simulink model "TorqueControl"  (R2022a)
settings: Solver=FixedStepAuto  StartTime=0.0  StopTime=inf  FixedStep=.001  RelTol=1e-3  EnableMultiTasking=on
undefined symbols (not defined in the file): DiscIntNeverNeededParam
libraries: simulink x7, slrealtimeutilitieslib x3, slrealtimeseriallib x2, slrealtimeloglib x2, eeGeneralControl x1
settings Model: sg_rtwmakecfg_data=_sg_IO75X_v1_2_0__sg_netxLib_MSVC140_  SimulationMode=external  ExtModeEnableFloating=off  Creator=a.beck  LastModifiedBy=Jason
settings SolverCC: ConcurrentTasks=on  AlgebraicLoopSolver=TrustRegion  PositivePriorityOrder=on  AutoInsertRateTranBlk=on  InsertRTBMode=Never (minimum delay)
settings DataIOCC: LimitDataPoints=on  SaveFormat=StructureWithTime  ReturnWorkspaceOutputs=off
settings OptimizationCC: BlockReduction=off  BooleanDataType=off  OptimizeBlockIOStorage=off  BufferReuse=off  GlobalBufferReuse=off  ExpressionFolding=off  LocalBlockOutputs=off  OptimizeDataStoreBuffers=off  BusAssignmentInplaceUpdate=off
settings DebuggingCC: SaveWithParameterizedLinksMsg=none  UnderspecifiedInitializationDetection=Classic  MergeDetectMultiDrivingBlocksExec=none  SignalResolutionControl=TryResolveAllWithWarning  TasksWithSamePriorityMsg=none  ParameterOverflowMsg=warning  UnconnectedInputMsg=warning  UnconnectedOutputMsg=warning  UnconnectedLineMsg=warning  SFUnexpectedBacktrackingDiag=warning  SFNoUnconditionalDefaultTransitionDiag=warning  SFExecutionAtInitializationDiag=none  SFMachineParentedDataDiag=warning  ArithmeticOperatorsInVariantConditions=warning
settings HardwareCC: ProdBitPerLong=64  ProdLongLongMode=on  ProdHWDeviceType=Intel->x86-64 (Linux 64)  TargetBitPerPointer=64  TargetBitPerSizeT=64  TargetBitPerPtrDiffT=64  TargetLongLongMode=on  TargetIntDivRoundTo=Zero  TargetEndianess=LittleEndian  TargetWordSize=64  TargetHWDeviceType=MATLAB Host
settings ModelReferenceCC: PropagateSignalLabelsOutOfModel=off
settings SFSimCC: SimUseLocalCustomCode=off  CustomCodeUndefinedFunction=UseInterfaceOnly
settings RTWCC: Description=Simulink Real-Time  SystemTargetFile=slrealtime.tlc  TemplateMakefile=slrealtime_default_tmf  RTWUseLocalCustomCode=off  Toolchain=Simulink Real-Time Toolchain  BuildConfiguration=Faster Runs  CodeExecutionProfiling=on  TargetLang=C++  DLArmComputeVersion=19.05
settings CodeAppCC: StateflowObjectComments=on
settings ConfigComp: CovMetricSettings=dw  CovSaveCumulativeToWorkspaceVar=on  CovSaveSingleToWorkspaceVar=on  CovExternalEMLEnable=off

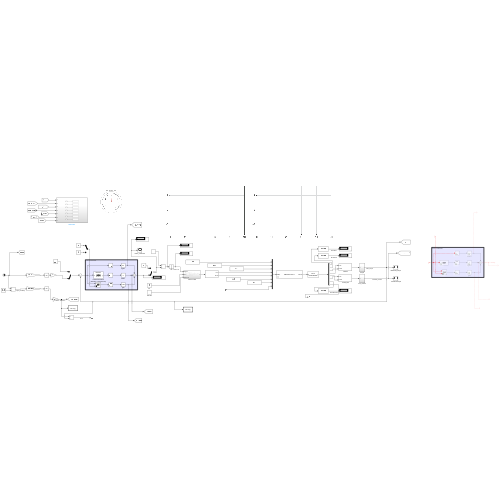
[thumbnail: Simulink's stored preview of the top-level diagram]
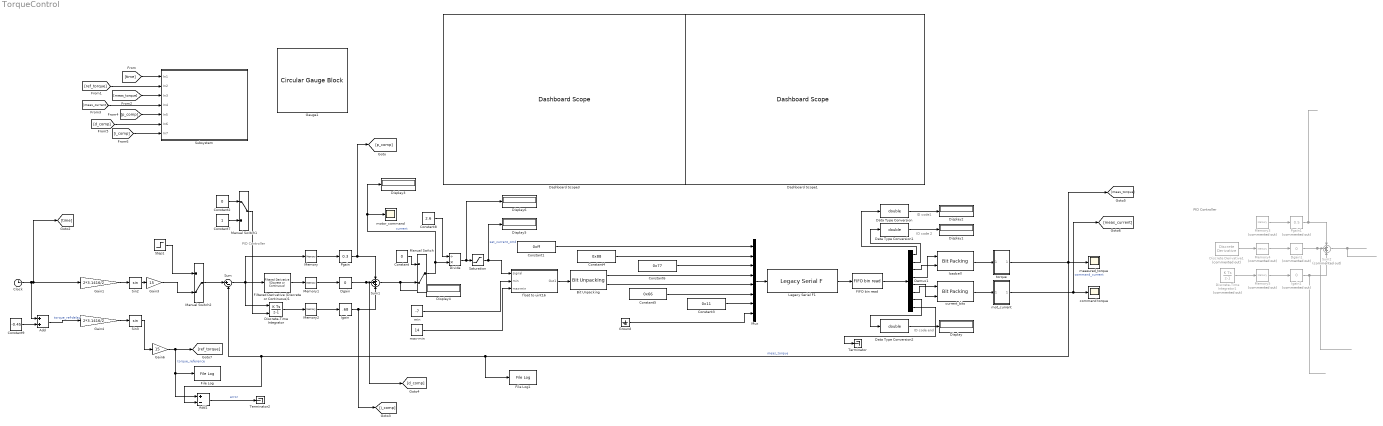
== system TorqueControl ==
  note: PID Controller
  note: ID code1
  note: ID code end
  note: ID code 2
  note: PID Controller
  Add : Sum
  Add1 : Sum  Inputs=+-
  Bit Unpacking : slrealtimeutilitieslib/Bit Unpacking  SignExtend=on  MaskBitPatterns={[0:7] [8:15]}  MaskPackDataType=uint16  MaskPackDataSize=[1]  MaskUnpackDataTypes={'uint8' 'uint8'}  MaskUnpackDataSizes={[1] [1]}
      settings: SourceProductBaseCode=XP
  Clock : Clock
  Constant : Constant  Value=0
  Constant1 : Constant  Value=0xff  VectorParams1D=off  OutDataTypeStr=uint8
  Constant2 : Constant  Value=0
  Constant3 : Constant  Value=0x11  VectorParams1D=off  OutDataTypeStr=uint8
  Constant4 : Constant  Value=0x88  VectorParams1D=off  OutDataTypeStr=uint8
  Constant5 : Constant  Value=0x66  VectorParams1D=off  OutDataTypeStr=uint8
  Constant6 : Constant  Value=0x77  VectorParams1D=off  OutDataTypeStr=uint8
  Constant7 : Constant
  Constant8 : Constant  Value=2.6
  Constant9 : Constant  Value=-0.45
  Dashboard Scope1 : DashboardScope  TimeSpan=50  Ymin=-5  Ymax=5
  Dashboard Scope3 : DashboardScope  TimeSpan=10  Ymin=-5  Ymax=5
  Data Type Conversion : DataTypeConversion  OutDataTypeStr=double  SaturateOnIntegerOverflow=off  RndMeth=Floor
  Data Type Conversion1 : DataTypeConversion  OutDataTypeStr=double  SaturateOnIntegerOverflow=off  RndMeth=Floor
  Data Type Conversion2 : DataTypeConversion  OutDataTypeStr=double  SaturateOnIntegerOverflow=off  RndMeth=Floor
  Demux1 : Demux  Outputs=8
  Dgain : simulink/Math Operations/Slider Gain  gain=0  low=0  high=50
  Dgain1 : simulink/Math Operations/Slider Gain  Commented=on  gain=0  low=0  high=50
  Discrete Derivative1 : simulink/Discrete/Discrete Derivative  Commented=on  gainval=1.0  ICPrevScaledInput=0.0  OutMin=[]  OutMax=[]  OutDataType=fixdt(1, 16)  OutScaling=2^-10  DoSatur=off
  Discrete-Time Integrator : DiscreteIntegrator  ExternalReset=rising  SampleTime=0.001  ICPrevOutput=DiscIntNeverNeededParam  ICPrevScaledInput=DiscIntNeverNeededParam
  Discrete-Time Integrator1 : DiscreteIntegrator  Commented=on  ExternalReset=rising  SampleTime=-1  ICPrevOutput=DiscIntNeverNeededParam  ICPrevScaledInput=DiscIntNeverNeededParam
  Display{,1..6} (7 alike) : Display
  Divide : Product  Inputs=/*
  FIFO bin read : slrealtimeseriallib/FIFO bin read  header={char([0xff, 0x88])}  lengths=[7]  hold=Hold last output if no new data  enable=off  maxsize=7  outputtype=8 bit uint null terminated  sampletime=-1
      settings: SourceProductBaseCode=XP
  File Log : slrealtimeloglib/File Log  decimation=1  inputProcessing=Elements as channels (sample based)
      settings: SourceProductBaseCode=XP
  File Log1 : slrealtimeloglib/File Log  decimation=1  inputProcessing=Elements as channels (sample based)
      settings: SourceProductBaseCode=XP
  Filtered Derivative (Discrete or Continuous)1 : eeGeneralControl/Filtered Derivative (Discrete or Continuous)  K=1  T=0.1  B=inf  A=-inf  minRatio=10  init_option=Inherited from block input  x0=0  Ts=-1
      settings: SourceProductBaseCode=PS
  Gain1 : Gain  Gain=2*3.1416/2
  Gain3 : Gain  Gain=15
  Gain4 : Gain  Gain=2*3.1416/2
  Gain6 : Gain  Gain=15
  Gauge1 : CircularGaugeBlock  ScaleMin=-5  ScaleMax=5
  Ground : Ground
  Igain : simulink/Math Operations/Slider Gain  gain=.68  low=0  high=50
  Igain1 : simulink/Math Operations/Slider Gain  Commented=on  gain=0  low=0  high=50
  Legacy Serial F1 : slrealtimeseriallib/Mainboard/Legacy Serial F  port=USB Serial Port 1  baud=115200  width=8  nstop=1  parity=None  ctsmode=off  fifosize=1024  idtype=8 bit uint null terminated  sampletime=0.01
      link override FIFO write: inputtype=8 bit uint null terminated
      link override Legacy Serial Read: dtype=8 bit uint null terminated
      link override Legacy Serial Write: dtype=8 bit uint null terminated
      settings: SourceProductBaseCode=XP
  Manual Switch : ManualSwitch  CurrentSetting=0
  Manual Switch1 : ManualSwitch
  Manual Switch2 : ManualSwitch  CurrentSetting=0
  Memory : Memory
  Memory1 : Memory
  Memory2 : Memory
  Memory3 : Memory  Commented=on
  Memory4 : Memory  Commented=on
  Memory5 : Memory  Commented=on
  Mux : Mux  Inputs=8
  Pgain : simulink/Math Operations/Slider Gain  gain=0.3  low=0  high=50
  Pgain1 : simulink/Math Operations/Slider Gain  Commented=on  gain=0.5  low=0  high=50
  Saturation : Saturate  UpperLimit=5  LowerLimit=-5
  Sin2 : Trigonometry
  Sin3 : Trigonometry
  Step1 : Step  Time=10  SampleTime=0
  Subsystem : Subsystem
  Sum : Sum  Inputs=|+-
  Sum1 : Sum  Inputs=+++
  Sum2 : Sum  Commented=on  Inputs=+++
  Terminator : Terminator
  Terminator2 : Terminator
  command torque : Scope
  current_bits : slrealtimeutilitieslib/Bit Packing  MaskBitPatterns={[0:7],[8:15]}  MaskPackDataType=uint16  MaskPackDataSize=[1]
      settings: SourceProductBaseCode=XP
  float to uint16 : Subsystem
  loadcell : slrealtimeutilitieslib/Bit Packing  MaskBitPatterns={[0:7],[8:15]}  MaskPackDataType=uint16  MaskPackDataSize=[1]
      settings: SourceProductBaseCode=XP
  max-min : Constant  Value=14  OutDataTypeStr=Inherit: Inherit via back propagation
  measured_torque : Scope
  min : Constant  Value=-7  OutDataTypeStr=Inherit: Inherit via back propagation
  mot_current : Subsystem
  motor_command : Scope
  torque : Subsystem
  wires:
  Constant1/1 -> Mux/1
  Mux/1 -> Legacy Serial F1/1
  Constant4/1 -> Mux/2
  Ground/1 -> Mux/8
  Constant3/1 -> Mux/7
  Bit Unpacking/1 -> Mux/4
  Bit Unpacking/2 -> Mux/5
  Constant6/1 -> Mux/3
  Constant5/1 -> Mux/6
  float to uint16/1(Out1) -> Bit Unpacking/1
  min/1 -> float to uint16/2(min)
  max-min/1 -> float to uint16/3(max-min)
  current_bits/1 -> mot_current/1(In1)
  Demux1/1 -> Data Type Conversion/1
  Demux1/2 -> Data Type Conversion1/1
  mot_current/1(Out1) -> command torque/1, [meas_current]  "command_current"
  Demux1/5 -> current_bits/2
  Data Type Conversion2/1 -> Display/1
  FIFO bin read/1 -> Demux1/1
  Demux1/8 -> Terminator/1
  Demux1/3 -> loadcell/2
  Demux1/4 -> loadcell/1
  loadcell/1 -> torque/1(In1)
  Data Type Conversion/1 -> Display2/1
  Legacy Serial F1/1 -> FIFO bin read/1
  Demux1/6 -> current_bits/1
  Data Type Conversion1/1 -> Display1/1
  Demux1/7 -> Data Type Conversion2/1
  Constant/1 -> Manual Switch/1
  Manual Switch/1 -> Divide/2, motor_command/1, Display3/1  "current"
  Saturation/1 -> Display5/1, float to uint16/1(signal)  "sat_current_cmd"
  Constant2/1 -> Manual Switch1/1
  Constant7/1 -> Manual Switch1/2
  Manual Switch1/1 -> Discrete-Time Integrator/2
  Pgain/1 -> [p_comp], Sum1/1
  Dgain/1 -> [d_comp], Sum1/2
  Igain/1 -> [i_comp], Sum1/3
  Filtered Derivative (Discrete or Continuous)1/1 -> Memory1/1
  Discrete-Time Integrator/1 -> Memory2/1
  Memory1/1 -> Dgain/1
  Sum/1 -> Filtered Derivative (Discrete or Continuous)1/1, Discrete-Time Integrator/1, Memory/1
  Memory/1 -> Pgain/1
  Memory2/1 -> Igain/1
  [time] -> Subsystem/1(In1)
  [meas_torque] -> Subsystem/3(In3)
  [ref_torque] -> Subsystem/2(In2)
  [meas_current] -> Subsystem/4(In4)
  [p_comp] -> Subsystem/5(In5)
  [d_comp] -> Subsystem/6(In6)
  [i_comp] -> Subsystem/7(In7)
  Clock/1 -> Gain1/1, [time], Add/1
  torque/1(Out1) -> File Log1/1, Add1/2, Sum/2, [meas_torque], measured_torque/1  "meas_torque"
  ? -> Discrete-Time Integrator1/2
  ? -> Discrete-Time Integrator1/1, Memory3/1, Discrete Derivative1/1
  Discrete-Time Integrator1/1 -> Memory5/1
  Memory4/1 -> Dgain1/1
  Memory5/1 -> Igain1/1
  Memory3/1 -> Pgain1/1
  Dgain1/1 -> Sum2/2
  Pgain1/1 -> Sum2/1
  Sum2/1 -> ?
  Igain1/1 -> Sum2/3
  Discrete Derivative1/1 -> Memory4/1
  Divide/1 -> Display6/1, Saturation/1
  Constant8/1 -> Divide/1
  Sin2/1 -> Gain3/1
  Gain1/1 -> Sin2/1
  Manual Switch2/1 -> Sum/1
  Step1/1 -> Manual Switch2/1
  Constant9/1 -> Add/2
  Gain4/1 -> Sin3/1
  Add/1 -> Gain4/1  "torque_ref-delay"
  Gain6/1 -> Add1/1, File Log/1, [ref_torque]  "torque_reference"
  Sin3/1 -> Gain6/1
  Gain3/1 -> Manual Switch2/2
  Add1/1 -> Terminator2/1  "error"
  Sum1/1 -> Display4/1, Manual Switch/2

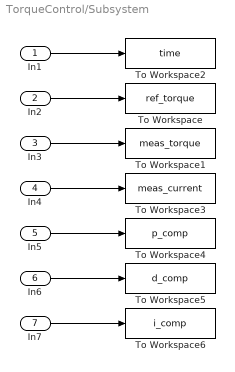
== system TorqueControl/Subsystem ==
  In1 : Inport
  In2 : Inport  Port=2
  In3 : Inport  Port=3
  In4 : Inport  Port=4
  In5 : Inport  Port=5
  In6 : Inport  Port=6
  In7 : Inport  Port=7
  To Workspace : ToWorkspace  VariableName=ref_torque  SaveFormat=Structure With Time  SampleTime=-1
  To Workspace1 : ToWorkspace  VariableName=meas_torque  SaveFormat=Structure With Time  SampleTime=-1
  To Workspace2 : ToWorkspace  VariableName=time  SaveFormat=Structure With Time  SampleTime=-1
  To Workspace3 : ToWorkspace  VariableName=meas_current  SaveFormat=Structure With Time  SampleTime=-1
  To Workspace4 : ToWorkspace  VariableName=p_comp  SaveFormat=Structure With Time  SampleTime=-1
  To Workspace5 : ToWorkspace  VariableName=d_comp  SaveFormat=Structure With Time  SampleTime=-1
  To Workspace6 : ToWorkspace  VariableName=i_comp  SaveFormat=Structure With Time  SampleTime=-1
  wires:
  In1/1 -> To Workspace2/1
  In3/1 -> To Workspace1/1
  In4/1 -> To Workspace3/1
  In5/1 -> To Workspace4/1
  In6/1 -> To Workspace5/1
  In7/1 -> To Workspace6/1
  In2/1 -> To Workspace/1

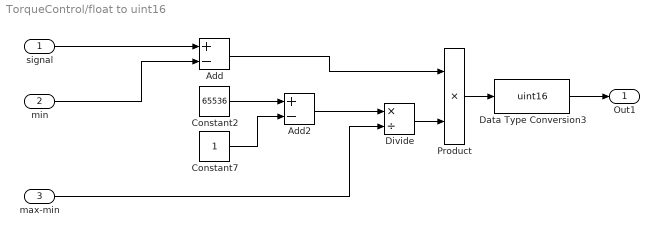
== system TorqueControl/float to uint16 ==
  signal : Inport
  min : Inport  Port=2
  max-min : Inport  Port=3
  Add : Sum  Inputs=+-
  Add2 : Sum  Inputs=+-
  Constant2 : Constant  Value=65536
  Constant7 : Constant  OutDataTypeStr=uint8
  Data Type Conversion3 : DataTypeConversion  OutDataTypeStr=uint16  SaturateOnIntegerOverflow=off  RndMeth=Floor
  Divide : Product  Inputs=*/
  Product : Product
  Out1 : Outport
  wires:
  Constant7/1 -> Add2/2
  Constant2/1 -> Add2/1
  min/1 -> Add/2
  Divide/1 -> Product/2
  Data Type Conversion3/1 -> Out1/1
  max-min/1 -> Divide/2
  Product/1 -> Data Type Conversion3/1
  signal/1 -> Add/1
  Add2/1 -> Divide/1
  Add/1 -> Product/1

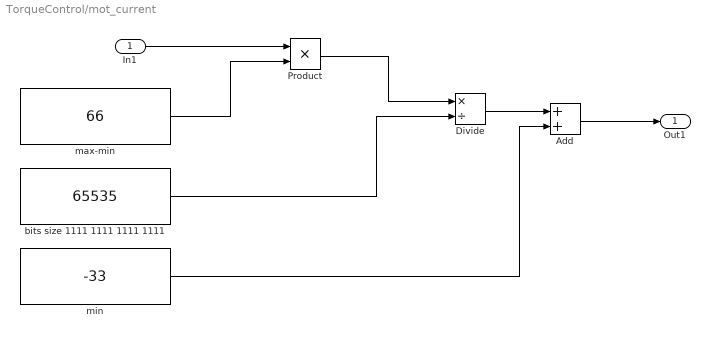
== system TorqueControl/mot_current ==
  In1 : Inport
  Add : Sum
  Divide : Product  Inputs=*/
  Product : Product
  bits size 1111 1111 1111 1111 : Constant  Value=65535
  max-min : Constant  Value=66
  min : Constant  Value=-33
  Out1 : Outport
  wires:
  bits size 1111 1111 1111 1111/1 -> Divide/2
  Divide/1 -> Add/1
  min/1 -> Add/2
  In1/1 -> Product/1
  Add/1 -> Out1/1
  max-min/1 -> Product/2
  Product/1 -> Divide/1

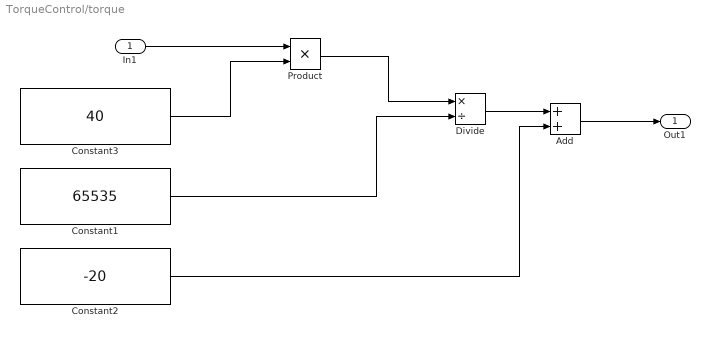
== system TorqueControl/torque ==
  In1 : Inport
  Add : Sum
  Constant1 : Constant  Value=65535
  Constant2 : Constant  Value=-20
  Constant3 : Constant  Value=40  OutDataTypeStr=uint8
  Divide : Product  Inputs=*/
  Product : Product
  Out1 : Outport
  wires:
  Constant1/1 -> Divide/2
  Divide/1 -> Add/1
  Constant2/1 -> Add/2
  In1/1 -> Product/1
  Add/1 -> Out1/1
  Constant3/1 -> Product/2
  Product/1 -> Divide/1
